simulink model "MCC"  (R2022b)
settings: Solver=ode23t  StartTime=0.0  StopTime=0.5  RelTol=1e-3
PreLoadFcn:
  | J = 0.28;
  | b = 8.5E-3;
  | C = 0;
  | Cr = 0;
  | K = 0.5093;
  | Ke = 0.5093;
  | Kt = 0.5093;
  | Kp = 100;
  | R = 0.13;
  | L = 1.6E-3;
  | U = 0;
  | E = 0;
  | theta = 0;
InitFcn:
  | TP2
libraries: slpidlib x1, simulink x1
settings Model: Creator=Youssef ABLALI  LastModifiedBy=Youssef ABLALI

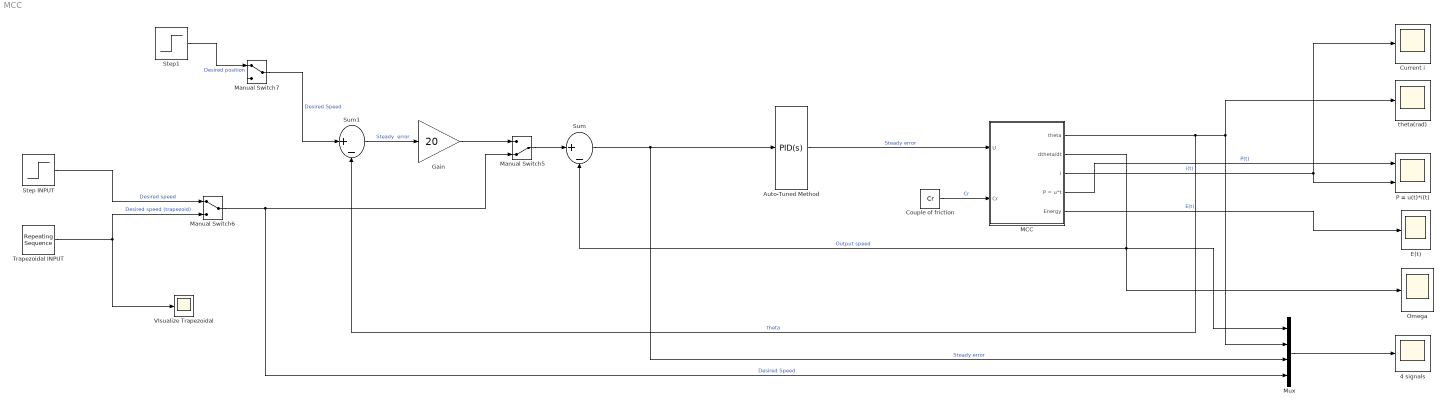
== system MCC ==
  4 signals : Scope
  "Auto-Tuned Method " : slpidlib/PID Controller  Controller=PID  Form=Parallel  TimeDomain=Continuous-time  UseExternalTs=off  SampleTime=-1  IntegratorMethod=Forward Euler  FilterMethod=Forward Euler  ControllerParametersSource=internal  P=4.548  I=17.8195536998464  UseKiTs=off  D=0.273504256839496  N=365.228401008731  UseFilter=on  TunerSelectOption=Transfer Function Based (PID Tuner App)  InitialConditionSource=internal  InitialConditionForIntegrator=0  InitialConditionForFilter=0  DifferentiatorICPrevScaledInput=0  ExternalReset=none  TrackingMode=off  Kt=1  LimitOutput=off  SatLimitsSource=internal  UpperSaturationLimit=inf  LowerSaturationLimit=-inf  LinearizeAsGain=on  AntiWindupMode=none  Kb=1  LimitIntegrator=off  UpperIntegratorSaturationLimit=inf  LowerIntegratorSaturationLimit=-inf  POutMin=[]  POutMax=[]  IOutMin=[]  IOutMax=[]  DOutMin=[]  DOutMax=[]  NOutMin=[]  NOutMax=[]  SumOutMin=[]  SumOutMax=[]  SaturationOutMin=[]  SaturationOutMax=[]  PParamMin=[]  PParamMax=[]  IParamMin=[]  IParamMax=[]  DParamMin=[]  DParamMax=[]  NParamMin=[]  NParamMax=[]  KbParamMin=[]  KbParamMax=[]  KtParamMin=[]  KtParamMax=[]  KbOutMin=[]  KbOutMax=[]  KtOutMin=[]  KtOutMax=[]  IntegratorOutMin=[]  IntegratorOutMax=[]  FilterOutMin=[]  FilterOutMax=[]  SumI1OutMin=[]  SumI1OutMax=[]  SumI2OutMin=[]  SumI2OutMax=[]  SumI3OutMin=[]  SumI3OutMax=[]  SumI4OutMin=[]  SumI4OutMax=[]  SumDOutMin=[]  SumDOutMax=[]  DifferentiatorOutMin=[]  DifferentiatorOutMax=[]  FilterDiffOutCoefMin=[]  FilterDiffOutCoefMax=[]  ReciprocalOutMin=[]  ReciprocalOutMax=[]  SumDenOutMin=[]  SumDenOutMax=[]  SumNumOutMin=[]  SumNumOutMax=[]  DivideOutMin=[]  DivideOutMax=[]  UdiffTsProdOutMin=[]  UdiffTsProdOutMax=[]  NTsProdOutMin=[]  NTsProdOutMax=[]  UintegralTsProdOutMin=[]  UintegralTsProdOutMax=[]  UngainTsProdOutMin=[]  UngainTsProdOutMax=[]  ClampingZeroOutDataTypeStr=Inherit: Inherit via back propagation  ClampingZeroOutMin=[]  ClampingZeroOutMax=[]  FilterDenConstantOutDataTypeStr=Inherit: Inherit via back propagation  FilterDenConstantOutMin=[]  FilterDenConstantOutMax=[]  PCopyOutDataTypeStr=Inherit: Inherit via back propagation  PCopyOutMin=[]  PCopyOutMax=[]  NCopyOutDataTypeStr=Inherit: Inherit via back propagation  NCopyOutMin=[]  NCopyOutMax=[]  IntegratorContinuousStateAttributes=''  IntegratorStateMustResolveToSignalObject=off  IntegratorRTWStateStorageClass=Auto  FilterContinuousStateAttributes=''  FilterStateMustResolveToSignalObject=off  FilterRTWStateStorageClass=Auto  ParallelPVariant=InternalParameters  IdealPVariant=Disabled  IVariant=InternalParameters  DVariant=InternalParameters  IntegratorVariant=Continuous  SatVariant=Disabled  AWVariant=Passthrough  PCopyVariant=Disabled  TRVariant=Disabled  FdbkBlocksVariant=Forward  IdealPFdbkVariant=Disabled  SatFdbkVariant=Disabled  DerivativeFilterVariant=ContFilter  NVariant=InternalParameters  NCopyVariant=Disabled  FilterICVariant=InternalICsFilter  IntegratorICVariant=InternalICs  ExternalResetVariant=Disabled  TRSumVariant=Passthrough  SumFdbkVariant=Disabled  SumVariant=Sum_PID  TsampFilterVariant=InternalTs  TsampNgainVariant=Passthrough  TsampIntegralVariant=Passthrough  ExternalSaturationOutDataTypeStr=Inherit: Same as second input
  Couple of friction : Constant  Value=Cr
  Current i : Scope
  E(t) : Scope
  Gain : Gain  Gain=20
  MCC : Subsystem
  Manual Switch5 : ManualSwitch  CurrentSetting=0
  Manual Switch6 : ManualSwitch
  Manual Switch7 : ManualSwitch
  Mux : Mux
  Omega : Scope
  P = u(t)*i(t) : Scope  NumInputPorts=2
  Step INPUT : Step  Time=0  SampleTime=0
  Step1 : Step  Time=0  SampleTime=0
  Sum : Sum  Inputs=|+-
  Sum1 : Sum  Inputs=|+-
  Trapezoidal INPUT : simulink/Sources/Repeating Sequence  rep_seq_t=[0 0.1 0.2 0.3 0.4 0.5]  rep_seq_y=[0 50 50 0 0 0]
  VIsualize Trapezoidal : Scope
  theta(rad) : Scope
  wires:
  Couple of friction/1 -> MCC/2(Cr)  "Cr"
  MCC/1(theta) -> Sum1/2, Mux/2, theta(rad)/1  "theta"
  Mux/1 -> 4 signals/1
  Sum/1 -> Mux/3, "Auto-Tuned Method "/1  "Steady error"
  "Auto-Tuned Method "/1 -> MCC/1(U)  "Steady error"
  MCC/2(dtheta/dt) -> Omega/1, Sum/2, Mux/1  "Output speed"
  Manual Switch5/1 -> Sum/1
  Sum1/1 -> Gain/1  "Steady  error"
  Gain/1 -> Manual Switch5/1
  MCC/3(i) -> Current i/1, P = u(t)*i(t)/2  "i(t)"
  Manual Switch6/1 -> Mux/4, Manual Switch5/2  "Desired Speed"
  Step INPUT/1 -> Manual Switch6/1  "Desired speed"
  Trapezoidal INPUT/1 -> VIsualize Trapezoidal/1, Manual Switch6/2  "Desired speed (trapezoid)"
  MCC/4(P = u*t) -> P = u(t)*i(t)/1  "P(t)"
  MCC/5(Energy) -> E(t)/1  "E(t)"
  Step1/1 -> Manual Switch7/1  "Desired position"
  Manual Switch7/1 -> Sum1/1  "Desired Speed"

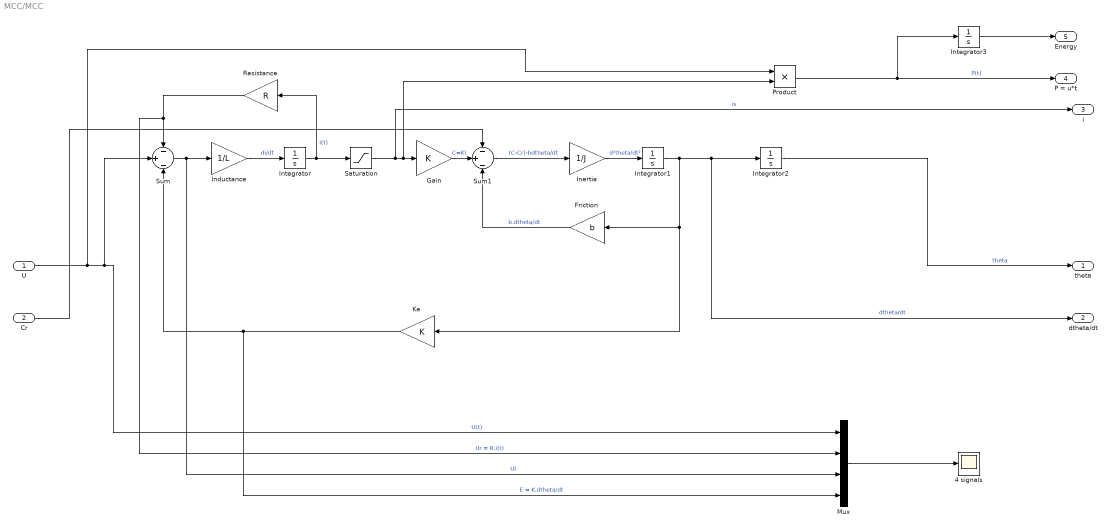
== system MCC/MCC ==
  U : Inport
  Cr : Inport  Port=2
  4 signals : Scope
  Friction : Gain  Gain=b
  Gain : Gain  Gain=K
  Inductance : Gain  Gain=1/L
  Inertia : Gain  Gain=1/J
  Integrator{,1..3} (4 alike) : Integrator
  Ke : Gain  Gain=K
  Mux : Mux
  Product : Product
  Resistance : Gain  Gain=R
  Saturation : Saturate  UpperLimit=20  LowerLimit=-20
  Sum : Sum  Inputs=-|+|-
  Sum1 : Sum  Inputs=-|+|-
  theta : Outport
  dtheta/dt : Outport  Port=2
  i : Outport  Port=3
  P = u*t : Outport  Port=4
  Energy : Outport  Port=5
  wires:
  Cr/1 -> Sum1/1
  Integrator1/1 -> Ke/1, Friction/1, dtheta/dt/1, Integrator2/1  "dtheta/dt"
  Ke/1 -> Mux/4, Sum/3  "E = K.dtheta/dt"
  Resistance/1 -> Mux/2, Sum/1  "Ur = R.i(t)"
  Gain/1 -> Sum1/2  "C=KI"
  Sum/1 -> Mux/3, Inductance/1  "Ul"
  Integrator2/1 -> theta/1  "theta"
  Sum1/1 -> Inertia/1  "(C-Cr)-bdtheta/dt"
  Friction/1 -> Sum1/3  "b.dtheta/dt"
  Inertia/1 -> Integrator1/1  "d²theta/dt²"
  Inductance/1 -> Integrator/1  "di/dt"
  Integrator/1 -> Saturation/1, Resistance/1  "i(t)"
  Mux/1 -> 4 signals/1
  Product/1 -> Integrator3/1, P = u*t/1  "P(t)"
  U/1 -> Product/1, Mux/1, Sum/2  "U(t)"
  Integrator3/1 -> Energy/1
  Saturation/1 -> i/1, Product/2, Gain/1  "is"
